simulink model "Demo3_model1"  (R2025b)
settings: Solver=VariableStepAuto  StartTime=0.0  StopTime=10.0  RelTol=1e-3
settings Model: Creator=FilipBabiec  LastModifiedBy=FilipBabiec

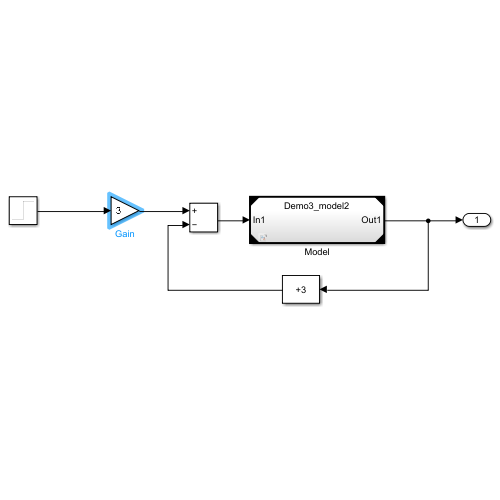
[thumbnail: Simulink's stored preview of the top-level diagram]
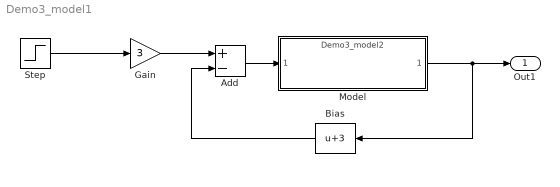
== system Demo3_model1 ==
  Add : Sum  Inputs=+-
  Bias : Bias  Bias=3  SaturateOnIntegerOverflow=off
  Gain : Gain  Gain=3
  Model : ModelReference  DisableCoverage=on  ModelNameDialog=Demo3_model2.slx  ModelReferenceVersion=1.2
  Step : Step  SampleTime=0
  Out1 : Outport
  wires:
  Step/1 -> Gain/1
  Model/1 -> Bias/1, Out1/1
  Gain/1 -> Add/1
  Add/1 -> Model/1
  Bias/1 -> Add/2
